simulink library "asmController_lib"  (R2018b)
settings: Solver=VariableStepAuto  StartTime=0.0  StopTime=10.0  RelTol=1e-3
undefined symbols (not defined in the file or in its folder): fswParams
libraries: Div_by_0_protection x1
settings Model: Creator=colem  LastModifiedBy=taylorreynolds

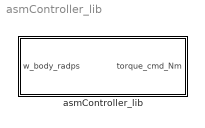
== system asmController_lib ==
  asmController_lib : Subsystem

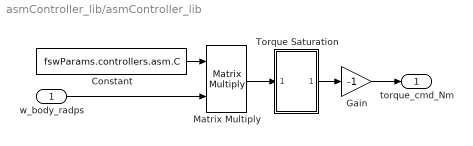
== system asmController_lib/asmController_lib ==
  w_body_radps : Inport
  Constant : Constant  Value=fswParams.controllers.asm.C
  Gain : Gain  Gain=-1
  Matrix Multiply : Product  Multiplication=Matrix(*)
  Torque Saturation : Subsystem
  torque_cmd_Nm : Outport
  wires:
  Constant/1 -> Matrix Multiply/1
  Torque Saturation/1(Out1) -> Gain/1
  Gain/1 -> torque_cmd_Nm/1
  Matrix Multiply/1 -> Torque Saturation/1(In1)
  w_body_radps/1 -> Matrix Multiply/2

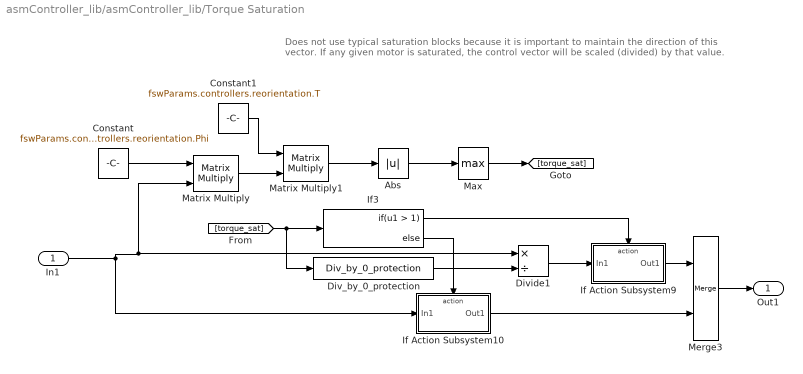
== system asmController_lib/asmController_lib/Torque Saturation ==
  note: Does not use typical saturation blocks because it is important to maintain the direction of this vector. If any given motor is saturated, the control vector will be scaled (divided) by that value.
  In1 : Inport
  Abs : Abs
  Constant : Constant  Value=fswParams.controllers.reorientation.Phi
  Constant1 : Constant  Value=fswParams.controllers.reorientation.T
  Div_by_0_protection : Div_by_0_protection/Div_by_0_protection  SystemSampleTime=-1
  Divide1 : Product  Inputs=*/
  If Action Subsystem10 : Subsystem  TreatAsAtomicUnit=on
  If Action Subsystem9 : Subsystem  TreatAsAtomicUnit=on
  If3 : If  IfExpression=u1 > 1
  Matrix Multiply : Product  Multiplication=Matrix(*)
  Matrix Multiply1 : Product  Multiplication=Matrix(*)
  Max : MinMax  Function=max
  Merge3 : Merge
  Out1 : Outport
  wires:
  If Action Subsystem9/1(Out1) -> Merge3/1
  If3/1 -> If Action Subsystem9/Action
  If3/2 -> If Action Subsystem10/Action
  If Action Subsystem10/1(Out1) -> Merge3/2
  Merge3/1 -> Out1/1
  Divide1/1 -> If Action Subsystem9/1(In1)
  Constant/1 -> Matrix Multiply/1
  In1/1 -> Matrix Multiply/2, Divide1/1, If Action Subsystem10/1(In1)
  Matrix Multiply/1 -> Matrix Multiply1/2
  Constant1/1 -> Matrix Multiply1/1
  Matrix Multiply1/1 -> Abs/1
  Abs/1 -> Max/1
  [torque_sat] -> Div_by_0_protection/1, If3/1
  Max/1 -> [torque_sat]
  Div_by_0_protection/1 -> Divide1/2

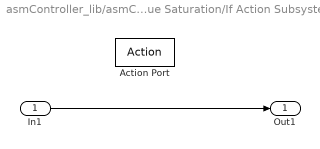
== system asmController_lib/asmController_lib/Torque Saturation/If Action Subsystem10 ==
  In1 : Inport
  Action Port : ActionPort
  Out1 : Outport
  wires:
  In1/1 -> Out1/1

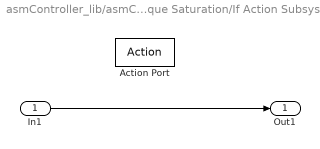
== system asmController_lib/asmController_lib/Torque Saturation/If Action Subsystem9 ==
  In1 : Inport
  Action Port : ActionPort
  Out1 : Outport
  wires:
  In1/1 -> Out1/1
